simulink model "graphical_function3_2018a"  (R2018a)
settings: Solver=FixedStepDiscrete  StartTime=0.0  StopTime=0.1  FixedStep=0.1  RelTol=1e-3  EnableMultiTasking=on
settings Model: Creator=bzhan  LastModifiedBy=86188
settings SolverCC: AutoInsertRateTranBlk=on
settings DataIOCC: LimitDataPoints=on  ReturnWorkspaceOutputs=on
settings OptimizationCC: LifeSpan=inf
settings DebuggingCC: AllowSymbolicDim=off  SFUnexpectedBacktrackingDiag=warning  SFNoUnconditionalDefaultTransitionDiag=warning  SFExecutionAtInitializationDiag=none
settings CodeAppCC: StateflowObjectComments=on
settings GRTTargetCC: TargetLangStandard=C89/C90 (ANSI)
settings ConfigComp: CovMetricSettings=dw  CovHtmlReporting=on  CovSaveCumulativeToWorkspaceVar=on  CovSaveSingleToWorkspaceVar=on  CovShowResultsExplorer=off  CovExternalEMLEnable=off  CovSFcnEnable=off

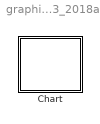
== system graphical_function3_2018a ==
  Chart : Stateflow chart  TreatAsAtomicUnit=on

== stateflow chart graphical_function3_2018a/Chart ==
  state index=find [function]
    (junction 2) -> (junction 12) [order 3] : {index=i;}
    (default) -> (junction 2) : {i=1;}
    (junction 2) -> (junction 10) [order 2] : [i>N]
    (junction 10) -> (junction 12) : {index=-1;}
    (junction 2) -> (junction 5) [order 1] : [i<=N&&a(i)==0]
    (junction 6) -> (junction 2)
    (junction 5) -> (junction 6) : {i=i+1;}
  state [an,rn]=get_acknack(wid,rid) [function]
    (default) -> (junction 30)
    (junction 30) -> (junction 33) : {an=buffer_acknack(rid,3)}
    (junction 33) -> (junction 34) : {rn=buffer_acknack(rid,4)}
  state B
    en: f("en_B");
    [acked_num(id),request_num(id)]=get_acknack(WriterId,id)
  state A
    en: f("en_A")
  (default) -> A
  A -> B : [find()==3]
  data: index function_output; wid function_input; rid function_input; an function_output; rn function_output; s function_input; a local =[0,0,1,2]; N local =4; WriterId local =1; id local =1; buffer_acknack local size=[2 4] =[1 1 1 1 ; 2 2 2 2]; acked_num local size=[1 2] =[0 0]; request_num local size=[1 3] =[0 0 0]
  function f(s):
    | function f(s)
    |   fprintf(s+"\n");
